simulink model "xor_ann_classifier"  (R2020a)
settings: Solver=VariableStepAuto  StartTime=0.0  StopTime=10.0  RelTol=1e-3
libraries: xbsIndex_r4 x41
settings Model: Creator=Bunny1719  LastModifiedBy=rhin1

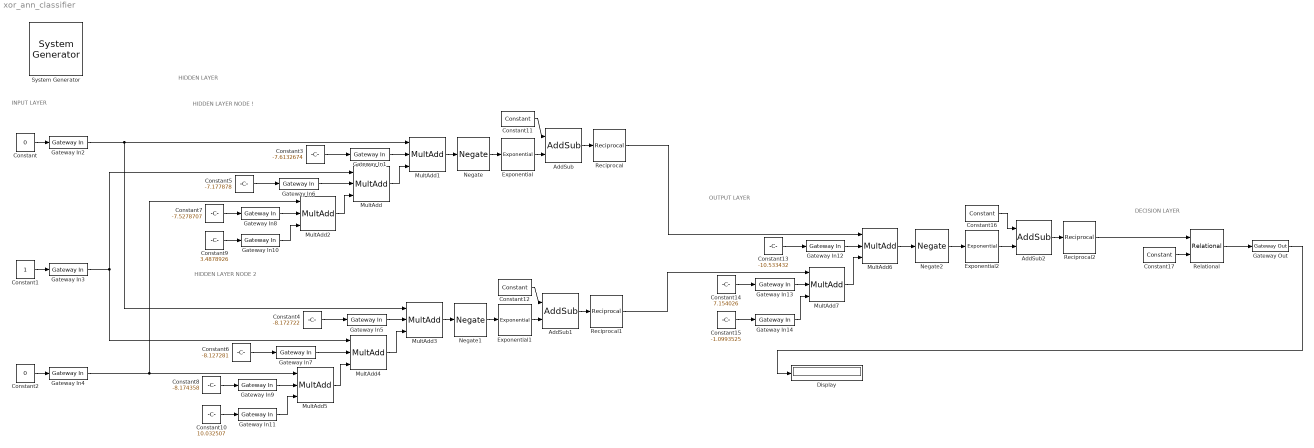
== system xor_ann_classifier ==
  note: HIDDEN LAYER
  note: DECISION LAYER
  note: OUTPUT LAYER
  note: INPUT LAYER
  note: HIDDEN LAYER NODE !
  note: HIDDEN LAYER NODE 2
  " System Generator" : xbsIndex_r4/ System Generator  Tag=genX  xilinxfamily=kintex7  part=xc7k325t  speed=-3  package=fbg676  synthesis_tool=Vivado  clock_wrapper=Clock Enables  directory=./netlist  proj_type=Vivado  Synth_file=Vivado Synthesis Defaults  Impl_file=Vivado Implementation Defaults  testbench=off  simulink_period=1  sysclk_period=10  dcm_input_clock_period=10  incr_netlist=off  trim_vbits=Everywhere in SubSystem  dbl_ovrd=According to Block Masks  core_generation=According to Block Masks  run_coregen=off  deprecated_control=off  eval_field=0  block_type=sysgen
  AddSub : xbsIndex_r4/AddSub  mode=Addition  use_carryin=off  use_carryout=off  en=off  latency=1  precision=Full  arith_type=Unsigned  n_bits=16  bin_pt=14  quantization=Truncate  overflow=Wrap  use_behavioral_HDL=off  hw_selection=Fabric  pipelined=off  dbl_ovrd=off  block_type=addsub
  AddSub1 : xbsIndex_r4/AddSub  mode=Addition  use_carryin=off  use_carryout=off  en=off  latency=1  precision=Full  arith_type=Unsigned  n_bits=16  bin_pt=14  quantization=Truncate  overflow=Wrap  use_behavioral_HDL=off  hw_selection=Fabric  pipelined=off  dbl_ovrd=off  block_type=addsub
  AddSub2 : xbsIndex_r4/AddSub  mode=Addition  use_carryin=off  use_carryout=off  en=off  latency=1  precision=Full  arith_type=Unsigned  n_bits=16  bin_pt=14  quantization=Truncate  overflow=Wrap  use_behavioral_HDL=off  hw_selection=Fabric  pipelined=off  dbl_ovrd=off  block_type=addsub
  Constant : Constant  Value=0
  Constant1 : Constant
  Constant10 : Constant  Value=10.032507
  Constant11 : xbsIndex_r4/Constant  const=1.0  gui_display_data_type=Floating-point  arith_type=Floating-point  n_bits=16  bin_pt=14  preci_type=Double  exp_width=8  frac_width=24  explicit_period=off  period=1  equ=P=C  opselect=C  inp2=PCIN>>17  opr=+  inp1=P  carry=CIN  dbl_ovrd=off  block_type=constant
  Constant12 : xbsIndex_r4/Constant  const=1.0  gui_display_data_type=Floating-point  arith_type=Floating-point  n_bits=16  bin_pt=14  preci_type=Double  exp_width=8  frac_width=24  explicit_period=off  period=1  equ=P=C  opselect=C  inp2=PCIN>>17  opr=+  inp1=P  carry=CIN  dbl_ovrd=off  block_type=constant
  Constant13 : Constant  Value=-10.533432
  Constant14 : Constant  Value=7.154026
  Constant15 : Constant  Value=-1.0993525
  Constant16 : xbsIndex_r4/Constant  const=1.0  gui_display_data_type=Floating-point  arith_type=Floating-point  n_bits=16  bin_pt=14  preci_type=Double  exp_width=8  frac_width=24  explicit_period=off  period=1  equ=P=C  opselect=C  inp2=PCIN>>17  opr=+  inp1=P  carry=CIN  dbl_ovrd=off  block_type=constant
  Constant17 : xbsIndex_r4/Constant  const=0.5  gui_display_data_type=Floating-point  arith_type=Floating-point  n_bits=16  bin_pt=14  preci_type=Double  exp_width=8  frac_width=24  explicit_period=off  period=1  equ=P=C  opselect=C  inp2=PCIN>>17  opr=+  inp1=P  carry=CIN  dbl_ovrd=off  block_type=constant
  Constant2 : Constant  Value=0
  Constant3 : Constant  Value=-7.6132674
  Constant4 : Constant  Value=-8.172722
  Constant5 : Constant  Value=-7.177878
  Constant6 : Constant  Value=-8.127281
  Constant7 : Constant  Value=-7.5278707
  Constant8 : Constant  Value=-8.174358
  Constant9 : Constant  Value=3.4878926
  Display : Display
  Exponential : xbsIndex_r4/Exponential  flow_control=NonBlocking  axi_optimize_goal=Resources  bmg_use=NoUsage  latency=1  has_a_tlast=off  has_a_tuser=off  en=off  has_result_tready=off  has_underflow=off  has_overflow=off  fpo_op_type=exponential  rate=1  has_b_tlast=false  has_b_tuser=false  result_tlast_behv=1  has_divide_by_zero=false  has_invalid_op=false  block_type=exponential
      settings: infoedit=Blocking: Wait for data on all inputs, allow back-pressure.<br>NonBlocking: operate every cycle in which all inputs are valid, no back-pressure.
  Exponential1 : xbsIndex_r4/Exponential  flow_control=NonBlocking  axi_optimize_goal=Resources  bmg_use=NoUsage  latency=1  has_a_tlast=off  has_a_tuser=off  en=off  has_result_tready=off  has_underflow=off  has_overflow=off  fpo_op_type=exponential  rate=1  has_b_tlast=false  has_b_tuser=false  result_tlast_behv=1  has_divide_by_zero=false  has_invalid_op=false  block_type=exponential
      settings: infoedit=Blocking: Wait for data on all inputs, allow back-pressure.<br>NonBlocking: operate every cycle in which all inputs are valid, no back-pressure.
  Exponential2 : xbsIndex_r4/Exponential  flow_control=NonBlocking  axi_optimize_goal=Resources  bmg_use=NoUsage  latency=1  has_a_tlast=off  has_a_tuser=off  en=off  has_result_tready=off  has_underflow=off  has_overflow=off  fpo_op_type=exponential  rate=1  has_b_tlast=false  has_b_tuser=false  result_tlast_behv=1  has_divide_by_zero=false  has_invalid_op=false  block_type=exponential
      settings: infoedit=Blocking: Wait for data on all inputs, allow back-pressure.<br>NonBlocking: operate every cycle in which all inputs are valid, no back-pressure.
  Gateway In{1..14} (14 alike) : xbsIndex_r4/Gateway In  gui_display_data_type=Floating-point  arith_type=Floating-point  n_bits=16  bin_pt=14  preci_type=Double  exp_width=8  frac_width=24  rows=1  columns=1  quantization="Round  (unbiased: +/- Inf)"  overflow=Saturate  period=1  UseAsADC=off  ADCChannel='1'  interface=None  automatic_assignment=on  address_offset=hex2dec('00')  intf_name=''  intf_description=''  default_value=0  timing_constraint=None  locs_specified=off  LOCs={}  io_standard={}  inherit_from_input=off  hdl_port=on  dbl_ovrd=off  block_type=gatewayin
  Gateway Out : xbsIndex_r4/Gateway Out  inherit_from_input=off  hdl_port=on  rows=1  columns=1  UseAsDAC=off  DACChannel='1'  interface=None  automatic_assignment=on  address_offset=hex2dec('00')  intf_name=''  intf_description=''  timing_constraint=None  locs_specified=off  LOCs={}  io_standard={}  block_type=gatewayout
  MultAdd{,1..7} (8 alike) : xbsIndex_r4/MultAdd  mode=Addition  en=off  infoeditControl=Fixed-point latency can be set to -1 or 0. The -1 selection will provide the optimum latency for max frequency for the given parameters.<br>Floating-point latency can be set to 0 or greater.  latency=0  precision=Full  arith_type=Unsigned  n_bits=16  bin_pt=14  block_type=multadd
  Negate : xbsIndex_r4/Negate  precision=Full  arith_type=Unsigned  n_bits=16  bin_pt=14  quantization=Truncate  overflow=Wrap  en=off  latency=1  dbl_ovrd=off  block_type=negate
  Negate1 : xbsIndex_r4/Negate  precision=Full  arith_type=Unsigned  n_bits=16  bin_pt=14  quantization=Truncate  overflow=Wrap  en=off  latency=1  dbl_ovrd=off  block_type=negate
  Negate2 : xbsIndex_r4/Negate  precision=Full  arith_type=Unsigned  n_bits=16  bin_pt=14  quantization=Truncate  overflow=Wrap  en=off  latency=1  dbl_ovrd=off  block_type=negate
  Reciprocal : xbsIndex_r4/Reciprocal  flow_control=NonBlocking  axi_optimize_goal=Resources  latency=1  has_a_tlast=off  has_a_tuser=off  en=off  has_result_tready=off  has_underflow=off  has_divide_by_zero=off  fpo_op_type=reciprocal  rate=1  has_b_tlast=false  has_b_tuser=false  result_tlast_behv=1  has_overflow=false  has_invalid_op=false  block_type=reciprocal
      settings: infoedit=Blocking: Wait for data on all inputs, allow back-pressure.<br>NonBlocking: operate every cycle in which all inputs are valid, no back-pressure.
  Reciprocal1 : xbsIndex_r4/Reciprocal  flow_control=NonBlocking  axi_optimize_goal=Resources  latency=1  has_a_tlast=off  has_a_tuser=off  en=off  has_result_tready=off  has_underflow=off  has_divide_by_zero=off  fpo_op_type=reciprocal  rate=1  has_b_tlast=false  has_b_tuser=false  result_tlast_behv=1  has_overflow=false  has_invalid_op=false  block_type=reciprocal
      settings: infoedit=Blocking: Wait for data on all inputs, allow back-pressure.<br>NonBlocking: operate every cycle in which all inputs are valid, no back-pressure.
  Reciprocal2 : xbsIndex_r4/Reciprocal  flow_control=NonBlocking  axi_optimize_goal=Resources  latency=1  has_a_tlast=off  has_a_tuser=off  en=off  has_result_tready=off  has_underflow=off  has_divide_by_zero=off  fpo_op_type=reciprocal  rate=1  has_b_tlast=false  has_b_tuser=false  result_tlast_behv=1  has_overflow=false  has_invalid_op=false  block_type=reciprocal
      settings: infoedit=Blocking: Wait for data on all inputs, allow back-pressure.<br>NonBlocking: operate every cycle in which all inputs are valid, no back-pressure.
  Relational : xbsIndex_r4/Relational  mode=a>=b  op_type=Bool  en=off  latency=1  dbl_ovrd=off  block_type=relational
  wires:
  Constant/1 -> Gateway In2/1
  Constant1/1 -> Gateway In3/1
  Constant2/1 -> Gateway In4/1
  Constant3/1 -> Gateway In1/1
  Constant4/1 -> Gateway In5/1
  Constant5/1 -> Gateway In6/1
  Constant6/1 -> Gateway In7/1
  Constant7/1 -> Gateway In8/1
  Constant8/1 -> Gateway In9/1
  Gateway In2/1 -> MultAdd1/1, MultAdd3/1
  Gateway In1/1 -> MultAdd1/2
  Gateway In3/1 -> MultAdd/1, MultAdd4/1
  Gateway In6/1 -> MultAdd/2
  Gateway In4/1 -> MultAdd2/1, MultAdd5/1
  Gateway In8/1 -> MultAdd2/2
  MultAdd/1 -> MultAdd1/3
  MultAdd2/1 -> MultAdd/3
  Constant9/1 -> Gateway In10/1
  Gateway In10/1 -> MultAdd2/3
  Gateway In5/1 -> MultAdd3/2
  MultAdd4/1 -> MultAdd3/3
  MultAdd5/1 -> MultAdd4/3
  Gateway In7/1 -> MultAdd4/2
  Gateway In9/1 -> MultAdd5/2
  Constant10/1 -> Gateway In11/1
  Gateway In11/1 -> MultAdd5/3
  Constant11/1 -> AddSub/1
  Exponential/1 -> AddSub/2
  Negate/1 -> Exponential/1
  MultAdd1/1 -> Negate/1
  AddSub/1 -> Reciprocal/1
  Negate1/1 -> Exponential1/1
  AddSub1/1 -> Reciprocal1/1
  Constant12/1 -> AddSub1/1
  Exponential1/1 -> AddSub1/2
  MultAdd3/1 -> Negate1/1
  Reciprocal/1 -> MultAdd6/1
  Constant13/1 -> Gateway In12/1
  Gateway In12/1 -> MultAdd6/2
  Constant14/1 -> Gateway In13/1
  Gateway In13/1 -> MultAdd7/2
  Reciprocal1/1 -> MultAdd7/1
  MultAdd7/1 -> MultAdd6/3
  Gateway In14/1 -> MultAdd7/3
  Constant15/1 -> Gateway In14/1
  MultAdd6/1 -> Negate2/1
  Constant16/1 -> AddSub2/1
  Negate2/1 -> Exponential2/1
  Exponential2/1 -> AddSub2/2
  AddSub2/1 -> Reciprocal2/1
  Gateway Out/1 -> Display/1
  Reciprocal2/1 -> Relational/1
  Constant17/1 -> Relational/2
  Relational/1 -> Gateway Out/1
